simulink model "P2_Ex9a"  (R2018a)
settings: Solver=VariableStepAuto  StartTime=0.0  StopTime=20  RelTol=1e-3
PreLoadFcn:
  | PreLoad_P2_Ex9_a
values from neighbouring files (symbols this model uses):
  Kp = 5    [PreLoad_P2_Ex9_b.m]
  Kt = 0.017    [PreLoad_P2_Ex9_b.m]
  Ts = 0.01    [PreLoad_P2_Ex9_b.m]
undefined symbols (not defined in the file or in its folder): K0, tau0
settings Model: Creator=Eneko Lerma  LastModifiedBy=Eneko Lerma

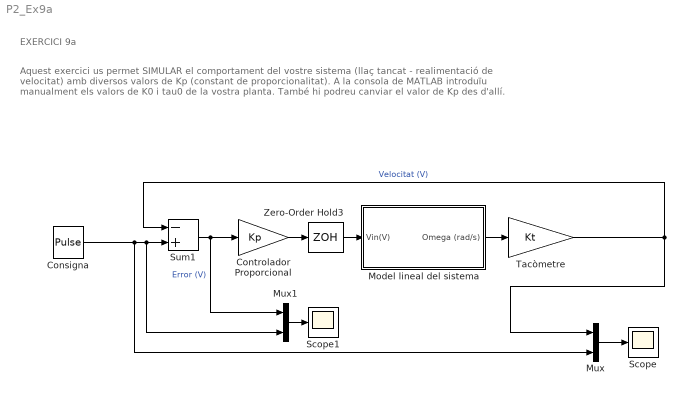
== system P2_Ex9a ==
  note: Aquest exercici us permet SIMULAR el comportament del vostre sistema (llaç tancat - realimentació de velocitat)
      | amb diversos valors de Kp (constant de proporcionalitat). A la consola de MATLAB introduïu manualment
      | els valors de K0 i tau0 de la vostra planta. També hi podreu canviar el valor de Kp des d'allí.
  note: EXERCICI 9a
  Consigna : DiscretePulseGenerator  PulseType=Time based  Period=5  PulseWidth=50
  Controlador Proporcional : Gain  Gain=Kp
  Model lineal del sistema : Subsystem
  Mux : Mux  Inputs=2
  Mux1 : Mux  Inputs=2
  Scope : Scope
  Scope1 : Scope
  Sum1 : Sum  Inputs=-+
  Tacòmetre : Gain  Gain=Kt
  Zero-Order Hold3 : ZeroOrderHold  SampleTime=Ts
  wires:
  Sum1/1 -> Mux1/1, Controlador Proporcional/1  "Error (V)"
  Consigna/1 -> Mux/2, Mux1/2, Sum1/2
  Tacòmetre/1 -> Mux/1, Sum1/1  "Velocitat (V)"
  Mux/1 -> Scope/1
  Controlador Proporcional/1 -> Zero-Order Hold3/1
  Model lineal del sistema/1(Omega (rad/s)) -> Tacòmetre/1
  Zero-Order Hold3/1 -> Model lineal del sistema/1(Vin(V))
  Mux1/1 -> Scope1/1

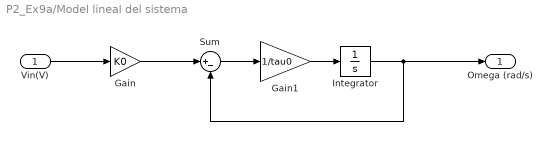
== system P2_Ex9a/Model lineal del sistema ==
  Vin(V) : Inport
  Gain : Gain  Gain=K0
  Gain1 : Gain  Gain=1/tau0
  Integrator : Integrator
  Sum : Sum  Inputs=|+-
  Omega (rad/s) : Outport
  wires:
  Integrator/1 -> Omega (rad/s)/1, Sum/2
  Sum/1 -> Gain1/1
  Vin(V)/1 -> Gain/1
  Gain1/1 -> Integrator/1
  Gain/1 -> Sum/1
